simulink model "Lab1_419_sim8"  (R2023b)
settings: Solver=VariableStepAuto  StartTime=0.0  StopTime=2  RelTol=1e-3
settings Model: Creator=Aiden  LastModifiedBy=Aiden

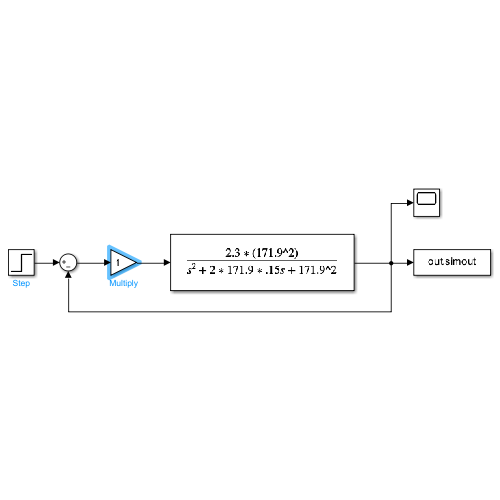
[thumbnail: Simulink's stored preview of the top-level diagram]
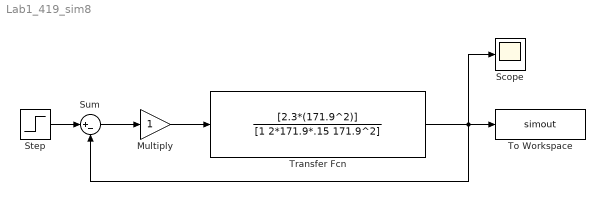
== system Lab1_419_sim8 ==
  Multiply : Gain
  Scope : Scope
  Step : Step  SampleTime=0
  Sum : Sum  Inputs=|+-
  To Workspace : ToWorkspace  VariableName=simout  SaveFormat=Timeseries  SampleTime=-1
  Transfer Fcn : TransferFcn  Numerator=[2.3*(171.9^2)]  Denominator=[1 2*171.9*.15 171.9^2]
  wires:
  Step/1 -> Sum/1
  Sum/1 -> Multiply/1
  Multiply/1 -> Transfer Fcn/1
  Transfer Fcn/1 -> Scope/1, Sum/2, To Workspace/1
